simulink model "Scattering_based_bis"  (R2020b)
settings: Solver=VariableStepAuto  StartTime=0.0  StopTime=10  RelTol=1e-3
values from neighbouring files (symbols this model uses):
  A = 1    [parameters_continous.m]
  b = 0.2    [parameters_continous.m]
  Be = 0    [parameters_continous.m]
  Bh = 70    [parameters_continous.m]
  Bm = 0.8    [parameters_continous.m]
  Bs = 0.8*4    (= 3.2)    [parameters_continous.m]
  Dh = 200    [parameters_continous.m]
  Dm = 0    [parameters_continous.m]
  Ds = 0    [parameters_continous.m]
  Fc = 1    [parameters_continous.m]
  Fip = 1    [parameters_continous.m]
  Je = 0    [parameters_continous.m]
  Jh = 0.5    [parameters_continous.m]
  Ke = 200    [parameters_continous.m]
  Kh = 2000    [parameters_continous.m]
  Km = 1    [parameters_continous.m]
  Ks = 4    [parameters_continous.m]
  Mm = 0.5    [parameters_continous.m]
  Ms = 2    [parameters_continous.m]
  Ph = 10000    [parameters_continous.m]
  tau = 100000    [parameters_continous.m]
settings Model: Creator=anuj  LastModifiedBy=Edoardo

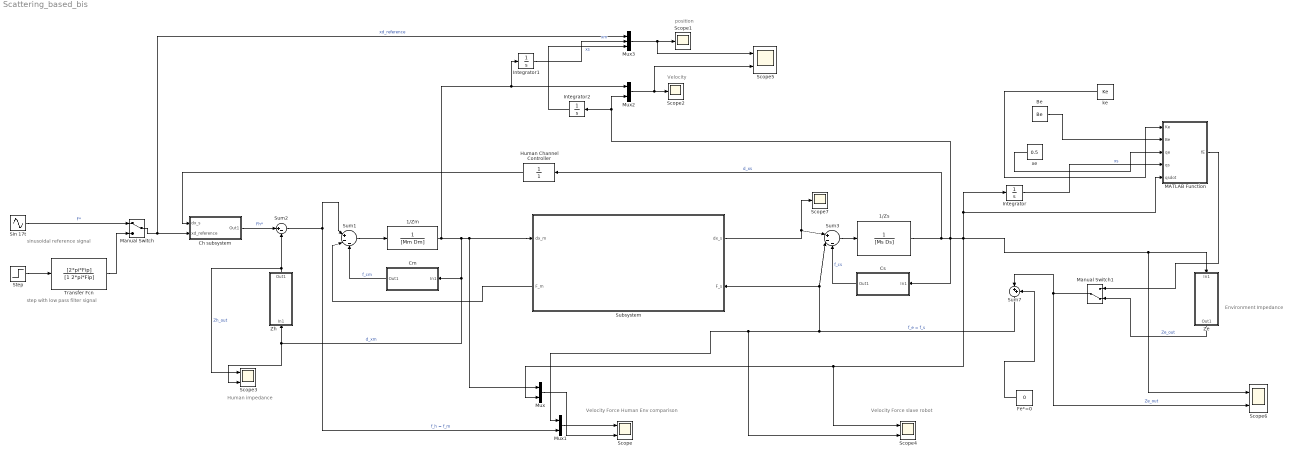
== system Scattering_based_bis ==
  note: Velocity
  note: position
  note: Environment Impedance
  note: Human impedance
  note: Velocity Force Human Env comparison
  note: Velocity Force slave robot
  note: sinusoidal reference signal
  note: step with low pass filter signal
  1/Zm : TransferFcn  Denominator=[Mm Dm]
  1/Zs : TransferFcn  Denominator=[Ms Ds]
  Be : Constant  Value=Be
  Ch subsystem : Subsystem
  Cm : Subsystem
  Cs : Subsystem
  Fe*=0 : Constant  Value=0
  Human Channel Controller : TransferFcn  Denominator=[1]
  Integrator : Integrator
  Integrator1 : Integrator
  Integrator2 : Integrator
  MATLAB Function : MATLAB Function  TreatAsAtomicUnit=on
  Manual Switch : ManualSwitch
  Manual Switch1 : ManualSwitch  CurrentSetting=0
  Mux : Mux  Inputs=2
  Mux1 : Mux  Inputs=2
  Mux2 : Mux  Inputs=2
  Mux3 : Mux  Inputs=3
  Scope{,3..6} (5 alike) : Scope  NumInputPorts=2
  Scope1 : Scope
  Scope2 : Scope
  Scope7 : Scope
  Sin 17t : Sin  Amplitude=A  Frequency=2*pi*Fc  SampleTime=0
  Step : Step  After=A  SampleTime=0
  Subsystem : Subsystem
      settings: PortSchema="{\"entries\":[{\"content\":{\"sides\":[{\"content\":{\"connectorIds\":[\"In1\",\"Out2\"]},\"type\":\"ConnectorPlacement.EquallySpacedRectSide\",\"uuid\":\"a4d8a1e6-493d-445f-9b62-4880423e0f65\"},{\"content\":{\"connectorIds\":[\"Out1\",\"In2\"],\"side\":\"RIGHT\"},\"type\":\"ConnectorPlacement.EquallySpacedRectSide\",\"uuid\":\"3d032ce1-a127-47bd-8907-4bd2e1f875d6\"},{\"content\":{\"connectorIds\":[],\"side\":\"TOP\"},\"type\":\"ConnectorPlacement.EquallySpacedRectSide\",\"uuid\":\"51a1971f-6e89-4837-8aa9-c8a237b527d1\"},{\"content\":{\"connectorIds\":[],\"side\":\"HIDDEN\"},\"type\":\"ConnectorPlacement.EquallySpacedRectSide\",\"uuid\":\"2bd12734-fa67-440d-bc97-b4fe58bfa138\"}]},\"type\":\"ConnectorPlacement.EquallySpacedConnector\",\"uuid\":\"cc0f3456-b5e1-4f18-b500-07b4336c0d17\"}],\"packageUris\":[\"http://schema.mathworks.com/mf0/Connector/R2020b\"],\"version\":\"1.0\"}"
  Sum1 : Sum  Inputs=|+--
  Sum2 : Sum  Inputs=|+-
  Sum3 : Sum  Inputs=|+--
  Sum7 : Sum  Inputs=|++
  Transfer Fcn : TransferFcn  Numerator=[2*pi*Fip]  Denominator=[1 2*pi*Fip]
  Ze : Subsystem
  Zh : Subsystem
  ke : Constant  Value=Ke
  xe : Constant  Value=0.5
  wires:
  Mux/1 -> Scope/2
  Mux1/1 -> Scope/1
  Sum2/1 -> Sum1/1, Mux1/2  "f_h = f_m"
  1/Zm/1 -> Integrator1/1, Mux2/1, Subsystem/1(dx_m), Mux/1, Zh/1(In1), Scope3/2, Cm/1(In1)  "d_xm"
  Sum1/1 -> 1/Zm/1
  Sum3/1 -> 1/Zs/1
  Fe*=0/1 -> Sum7/2
  Sum7/1 -> Mux1/1, Scope4/2, Subsystem/2(F_s), Sum3/2  "f_e = f_s"
  Ch subsystem/1(Out1) -> Sum2/1  "Fh*"
  Be/1 -> MATLAB Function/2(Be)
  xe/1 -> MATLAB Function/3(qe)
  ke/1 -> MATLAB Function/1(Ke)
  Integrator/1 -> MATLAB Function/4(qs)  "xs"
  Transfer Fcn/1 -> Manual Switch/2
  Step/1 -> Transfer Fcn/1
  Human Channel Controller/1 -> Ch subsystem/1(dx_s)
  Manual Switch/1 -> Mux3/1, Ch subsystem/2(xd_reference)  "xd_reference"
  Sin 17t/1 -> Manual Switch/1  "F*"
  MATLAB Function/1(fE) -> Manual Switch1/1
  1/Zs/1 -> Cs/1(In1), Mux/2, Scope4/1, MATLAB Function/5(qsdot), Integrator/1, Scope6/1, Ze/1(In1), Integrator2/1, Mux2/2, Human Channel Controller/1  "d_xs"
  Manual Switch1/1 -> Scope6/2, Sum7/1  "Ze_out"
  Zh/1(Out1) -> Sum2/2, Scope3/1  "Zh_out"
  Cm/1(Out1) -> Sum1/3  "f_cm"
  Ze/1(Out1) -> Manual Switch1/2  "Ze_out"
  Integrator1/1 -> Mux3/2  "xm"
  Integrator2/1 -> Mux3/3  "xs"
  Mux2/1 -> Scope2/1, Scope5/2
  Mux3/1 -> Scope1/1, Scope5/1
  Subsystem/2(F_m) -> Sum1/2
  Subsystem/1(dx_s) -> Scope7/1, Sum3/1
  Cs/1(Out1) -> Sum3/3  "f_cs"

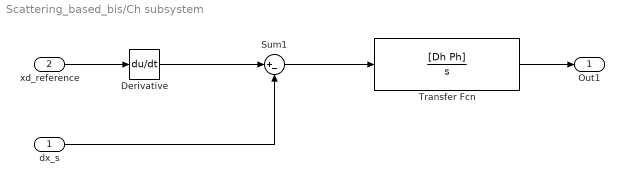
== system Scattering_based_bis/Ch subsystem ==
  dx_s : Inport
  xd_reference : Inport  Port=2
  Derivative : Derivative
  Sum1 : Sum  Inputs=|+-
  Transfer Fcn : TransferFcn  Numerator=[Dh Ph]  Denominator=[1 0]
  Out1 : Outport
  wires:
  dx_s/1 -> Sum1/2
  Sum1/1 -> Transfer Fcn/1
  xd_reference/1 -> Derivative/1
  Derivative/1 -> Sum1/1
  Transfer Fcn/1 -> Out1/1

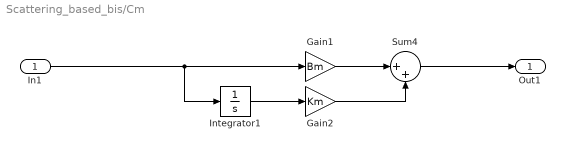
== system Scattering_based_bis/Cm ==
  In1 : Inport
  Gain1 : Gain  Gain=Bm
  Gain2 : Gain  Gain=Km
  Integrator1 : Integrator
  Sum4 : Sum  Inputs=|++
  Out1 : Outport
  wires:
  Sum4/1 -> Out1/1
  Gain1/1 -> Sum4/1
  Integrator1/1 -> Gain2/1
  In1/1 -> Gain1/1, Integrator1/1
  Gain2/1 -> Sum4/2

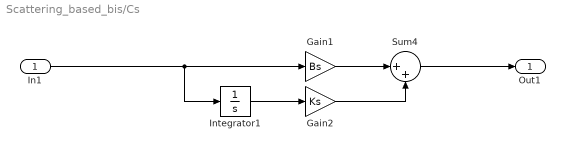
== system Scattering_based_bis/Cs ==
  In1 : Inport
  Gain1 : Gain  Gain=Bs
  Gain2 : Gain  Gain=Ks
  Integrator1 : Integrator
  Sum4 : Sum  Inputs=|++
  Out1 : Outport
  wires:
  Sum4/1 -> Out1/1
  Gain1/1 -> Sum4/1
  Integrator1/1 -> Gain2/1
  In1/1 -> Gain1/1, Integrator1/1
  Gain2/1 -> Sum4/2

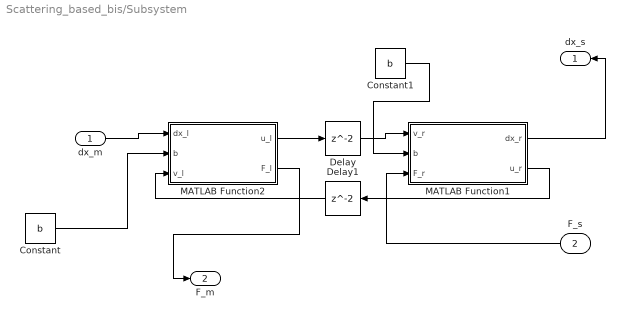
== system Scattering_based_bis/Subsystem ==
  dx_m : Inport
  F_s : Inport  Port=2
  Constant : Constant  Value=b
  Constant1 : Constant  Value=b
  Delay : Delay
  Delay1 : Delay
  MATLAB Function1 : MATLAB Function  TreatAsAtomicUnit=on
  MATLAB Function2 : MATLAB Function  TreatAsAtomicUnit=on
  dx_s : Outport
  F_m : Outport  Port=2
  wires:
  dx_m/1 -> MATLAB Function2/1(dx_l)
  MATLAB Function2/2(F_l) -> F_m/1
  MATLAB Function2/1(u_l) -> Delay/1
  Delay/1 -> MATLAB Function1/1(v_r)
  Delay1/1 -> MATLAB Function2/3(v_l)
  MATLAB Function1/2(u_r) -> Delay1/1
  MATLAB Function1/1(dx_r) -> dx_s/1
  F_s/1 -> MATLAB Function1/3(F_r)
  Constant/1 -> MATLAB Function2/2(b)
  Constant1/1 -> MATLAB Function1/2(b)

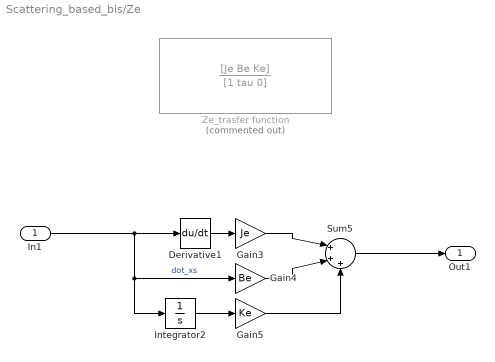
== system Scattering_based_bis/Ze ==
  In1 : Inport
  Derivative1 : Derivative
  Gain3 : Gain  Gain=Je
  Gain4 : Gain  Gain=Be
  Gain5 : Gain  Gain=Ke
  Integrator2 : Integrator
  Sum5 : Sum  Inputs=|+++
  Ze_trasfer function : TransferFcn  Commented=on  Numerator=[Je Be Ke]  Denominator=[1 tau 0]
  Out1 : Outport
  wires:
  Gain4/1 -> Sum5/2
  Gain3/1 -> Sum5/1
  Gain5/1 -> Sum5/3
  Sum5/1 -> Out1/1
  Integrator2/1 -> Gain5/1
  In1/1 -> Integrator2/1, Gain4/1, Derivative1/1  "dot_xs"
  Derivative1/1 -> Gain3/1

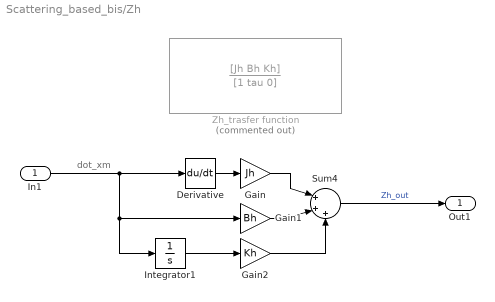
== system Scattering_based_bis/Zh ==
  note: dot_xm
  In1 : Inport
  Derivative : Derivative
  Gain : Gain  Gain=Jh
  Gain1 : Gain  Gain=Bh
  Gain2 : Gain  Gain=Kh
  Integrator1 : Integrator
  Sum4 : Sum  Inputs=|+++
  Zh_trasfer function : TransferFcn  Commented=on  Numerator=[Jh Bh Kh]  Denominator=[1 tau 0]
  Out1 : Outport
  wires:
  Derivative/1 -> Gain/1
  Integrator1/1 -> Gain2/1
  Gain2/1 -> Sum4/3
  Gain1/1 -> Sum4/2
  Gain/1 -> Sum4/1
  Sum4/1 -> Out1/1  "Zh_out"
  In1/1 -> Gain1/1, Integrator1/1, Derivative/1

== matlab function Scattering_based_bis/Subsystem/MATLAB Function2 ==
  data: dx_l input; b input; u_l output; v_l input; F_l output
function [u_l, F_l] = left(dx_l, b, v_l)

u_l = sqrt(2*b)*dx_l + v_l;
F_l = b*dx_l + sqrt(2*b)*v_l;

== matlab function Scattering_based_bis/MATLAB Function ==
  data: Ke input; fE output; Be input; qe input; qs input; qsdot input
function fE = environment(Ke, Be, qe, qs, qsdot)
    if qs > qe
        fE = Ke * (qs - qe) + Be * qsdot;
    else
        fE = 0;
    end
end

== matlab function Scattering_based_bis/Subsystem/MATLAB Function1 ==
  data: v_r input; b input; dx_r output; F_r input; u_r output
function [dx_r, u_r] = right(v_r, b, F_r)

u_r  = sqrt(2/b)*F_r - v_r;
dx_r = -(1/b)*(F_r - sqrt(2*b)*v_r);
